simulink model "IIR"  (R2018b)
settings: Solver=VariableStepAuto  StartTime=0.0  StopTime=10.0  RelTol=1e-3
libraries: dspsrcs4 x2
settings Model: Creator=MrGoshak  LastModifiedBy=MrGoshak

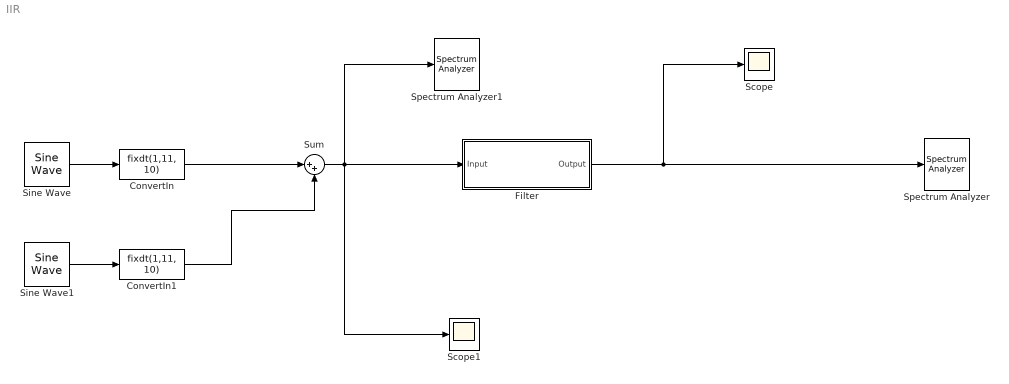
== system IIR ==
  ConvertIn : DataTypeConversion  OutDataTypeStr=fixdt(1,11, 10)  RndMeth=Nearest  SaturateOnIntegerOverflow=on
  ConvertIn1 : DataTypeConversion  OutDataTypeStr=fixdt(1,11, 10)  RndMeth=Nearest  SaturateOnIntegerOverflow=on
  Filter : Subsystem  Tag=FilterWizardSubSystem
      settings: ErrorFcn=dspFilterRealizedInBasicElemsAlgLoopErrFcnCallback
  Scope : Scope
  Scope1 : Scope
  Sine Wave : dspsrcs4/Sine Wave  Amplitude=1/2  Frequency=10000  Phase=0  SampleMode=Discrete  OutComplex=Real  CompMethod=Trigonometric fcn  TableSize=Speed  SampleTime=1/500000  SamplesPerFrame=1  ResetState=Restart at time zero  OutputFrames=off  dataType=double  wordLen=16  udDataType=sfix(16)  fracBitsMode=Best precision  numFracBits=15  OutDataTypeStr=double  LastOutDataTypeStr=double
  Sine Wave1 : dspsrcs4/Sine Wave  Amplitude=1/2  Frequency=60000  Phase=0  SampleMode=Discrete  OutComplex=Real  CompMethod=Trigonometric fcn  TableSize=Speed  SampleTime=1/500000  SamplesPerFrame=1  ResetState=Restart at time zero  OutputFrames=off  dataType=double  wordLen=16  udDataType=sfix(16)  fracBitsMode=Best precision  numFracBits=15  OutDataTypeStr=double  LastOutDataTypeStr=double
  Spectrum Analyzer : SpectrumAnalyzer
  Spectrum Analyzer1 : SpectrumAnalyzer
  Sum : Sum  Inputs=|++  OutDataTypeStr=fixdt(1,12, 11)  SaturateOnIntegerOverflow=on  InputSameDT=on
  wires:
  Sine Wave/1 -> ConvertIn/1
  ConvertIn1/1 -> Sum/2
  Sine Wave1/1 -> ConvertIn1/1
  Sum/1 -> Filter/1(Input), Spectrum Analyzer1/1, Scope1/1
  ConvertIn/1 -> Sum/1
  Filter/1(Output) -> Scope/1, Spectrum Analyzer/1

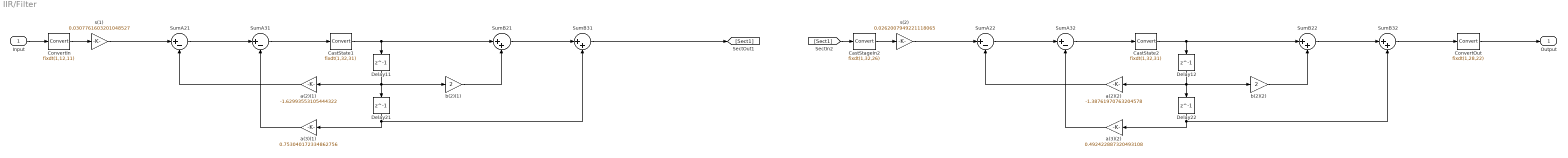
== system IIR/Filter ==
  Input : Inport
  CastStageIn2 : DataTypeConversion  OutDataTypeStr=fixdt(1,32,26)  SaturateOnIntegerOverflow=on
  CastState1 : DataTypeConversion  OutDataTypeStr=fixdt(1,32,31)  SaturateOnIntegerOverflow=on
  CastState2 : DataTypeConversion  OutDataTypeStr=fixdt(1,32,31)  SaturateOnIntegerOverflow=on
  ConvertIn : DataTypeConversion  OutDataTypeStr=fixdt(1,12,11)  RndMeth=Nearest  SaturateOnIntegerOverflow=on
  ConvertOut : DataTypeConversion  OutDataTypeStr=fixdt(1,28,22)  SaturateOnIntegerOverflow=on
  Delay{11..12,21..22} (4 alike) : Delay  DelayLength=1  InitialCondition=0
  SumA{21..22,31..32} (4 alike) : Sum  Inputs=|+-  AccumDataTypeStr=fixdt(1,40,35)  OutDataTypeStr=fixdt(1,40,35)  SaturateOnIntegerOverflow=on
  SumB{21..22,31..32} (4 alike) : Sum  Inputs=|++  AccumDataTypeStr=fixdt(1,40,34)  OutDataTypeStr=fixdt(1,40,34)  SaturateOnIntegerOverflow=on
  a(2)(1) : Gain  Gain=-1.62993553105444322  ParamDataTypeStr=fixdt(1,16,14)  OutDataTypeStr=fixdt(1,48,45)  SaturateOnIntegerOverflow=on
  a(2)(2) : Gain  Gain=-1.38761970763204578  ParamDataTypeStr=fixdt(1,16,14)  OutDataTypeStr=fixdt(1,48,45)  SaturateOnIntegerOverflow=on
  a(3)(1) : Gain  Gain=0.753040172334862756  ParamDataTypeStr=fixdt(1,16,14)  OutDataTypeStr=fixdt(1,48,45)  SaturateOnIntegerOverflow=on
  a(3)(2) : Gain  Gain=0.492422887320493108  ParamDataTypeStr=fixdt(1,16,14)  OutDataTypeStr=fixdt(1,48,45)  SaturateOnIntegerOverflow=on
  b(2)(1) : Gain  Gain=2  ParamDataTypeStr=fixdt(1,16,13)  OutDataTypeStr=fixdt(1,48,44)  SaturateOnIntegerOverflow=on
  b(2)(2) : Gain  Gain=2  ParamDataTypeStr=fixdt(1,16,13)  OutDataTypeStr=fixdt(1,48,44)  SaturateOnIntegerOverflow=on
  s(1) : Gain  Gain=0.0307761603201048527  ParamDataTypeStr=fixdt(1,16,20)  OutDataTypeStr=fixdt(1,32,30)  SaturateOnIntegerOverflow=on
  s(2) : Gain  Gain=0.0262007949221118065  ParamDataTypeStr=fixdt(1,16,20)  OutDataTypeStr=fixdt(1,32,30)  SaturateOnIntegerOverflow=on
  Output : Outport
  wires:
  Input/1 -> ConvertIn/1
  s(1)/1 -> SumA21/1
  SumA21/1 -> SumA31/1
  SumA31/1 -> CastState1/1
  CastState1/1 -> SumB21/1, Delay11/1
  SumB21/1 -> SumB31/1
  SumB31/1 -> [Sect1]
  a(2)(1)/1 -> SumA21/2
  Delay11/1 -> a(2)(1)/1, b(2)(1)/1, Delay21/1
  b(2)(1)/1 -> SumB21/2
  a(3)(1)/1 -> SumA31/2
  Delay21/1 -> a(3)(1)/1, SumB31/2
  ConvertIn/1 -> s(1)/1
  [Sect1] -> CastStageIn2/1
  s(2)/1 -> SumA22/1
  SumA22/1 -> SumA32/1
  SumA32/1 -> CastState2/1
  CastState2/1 -> SumB22/1, Delay12/1
  SumB22/1 -> SumB32/1
  SumB32/1 -> ConvertOut/1
  a(2)(2)/1 -> SumA22/2
  Delay12/1 -> a(2)(2)/1, b(2)(2)/1, Delay22/1
  b(2)(2)/1 -> SumB22/2
  a(3)(2)/1 -> SumA32/2
  Delay22/1 -> a(3)(2)/1, SumB32/2
  ConvertOut/1 -> Output/1
  CastStageIn2/1 -> s(2)/1
